simulink model "EKF_model"  (R2021b)
settings: Solver=VariableStepAuto  StartTime=0.0  StopTime=10.0  RelTol=1e-3
values from neighbouring files (symbols this model uses):
  Ts = 0.04    [EKF_simulation.m]
settings Model: Creator=jcwon  LastModifiedBy=jcwon

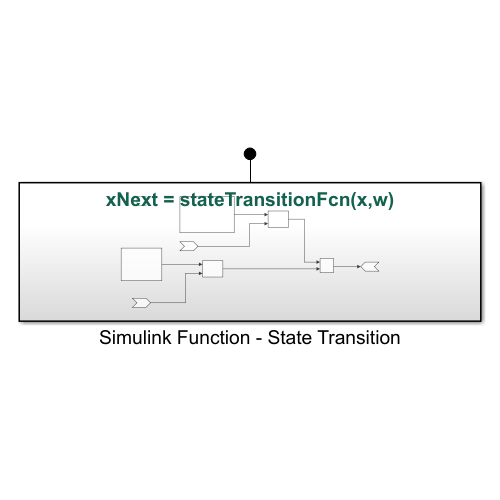
[thumbnail: Simulink's stored preview of the top-level diagram]
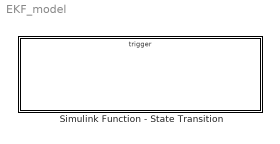
== system EKF_model ==
  Simulink Function - State Transition : Subsystem  TreatAsAtomicUnit=on

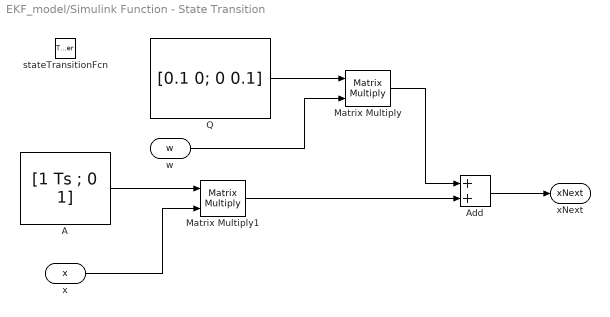
== system EKF_model/Simulink Function - State Transition ==
  stateTransitionFcn : TriggerPort  TriggerType=function-call  IsSimulinkFunction=on  FunctionName=stateTransitionFcn  FunctionVisibility=scoped  VariantControl=(inherit)
  A : Constant  Value=[1 Ts ; 0 1]
  Add : Sum
  Matrix Multiply : Product  Multiplication=Matrix(*)
  Matrix Multiply1 : Product  Multiplication=Matrix(*)
  Q : Constant  Value=[0.1 0; 0 0.1]
  x : ArgIn  DisableCoverage=on  ArgumentName=x
  w : ArgIn  Port=2  ArgumentName=w
  xNext : ArgOut  DisableCoverage=on  ArgumentName=xNext
  wires:
  w/1 -> Matrix Multiply/2
  x/1 -> Matrix Multiply1/2
  Q/1 -> Matrix Multiply/1
  A/1 -> Matrix Multiply1/1
  Add/1 -> xNext/1
  Matrix Multiply1/1 -> Add/2
  Matrix Multiply/1 -> Add/1
